simulink model "PIL_lqr_nl"  (R2024b)
settings: Solver=VariableStepAuto  StartTime=0.0  StopTime=params.simtime  RelTol=1e-3
values from neighbouring files (symbols this model uses):
  params = parameters()    [lqr_compare.m]    (also in lqr_main_isolated.m; lqr_pil.m)
undefined symbols (not defined in the file or in its folder): CR, LF, nl_model
libraries: instrumentseriallib x12
settings Model: Creator=ben83  LastModifiedBy=ben
settings RTWCC: GPUComputeCapability=3.5

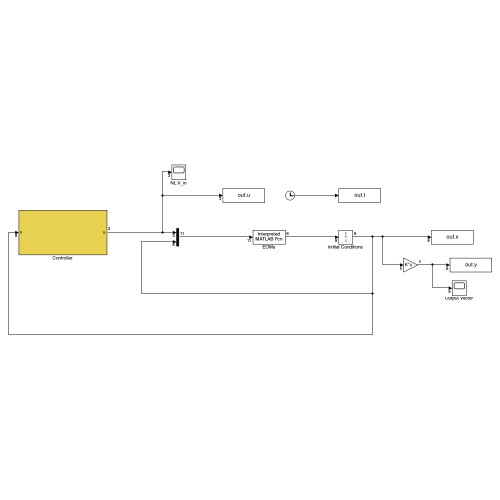
[thumbnail: Simulink's stored preview of the top-level diagram]
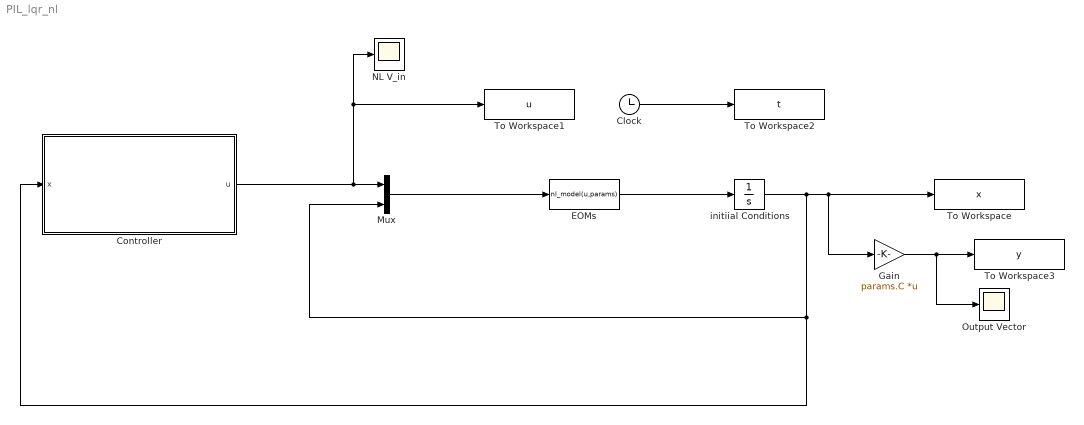
== system PIL_lqr_nl ==
  Clock : Clock
  Controller : Subsystem
  EOMs : MATLABFcn  MATLABFcn=nl_model(u,params)  OutputDimensions=8
  Gain : Gain  Gain=params.C  Multiplication=Matrix(K*u)
  Mux : Mux  Inputs=2
  NL V_in : Scope
  Output Vector : Scope
  To Workspace : ToWorkspace  VariableName=x  SampleTime=-1
  To Workspace1 : ToWorkspace  VariableName=u  SampleTime=-1
  To Workspace2 : ToWorkspace  VariableName=t  SampleTime=-1
  To Workspace3 : ToWorkspace  VariableName=y  SampleTime=-1
  initiial Conditions : Integrator  InitialCondition=params.ic
  wires:
  EOMs/1 -> initiial Conditions/1
  Mux/1 -> EOMs/1
  Clock/1 -> To Workspace2/1
  Controller/1(u) -> NL V_in/1, To Workspace1/1, Mux/1
  initiial Conditions/1 -> Controller/1(x), Mux/2, Gain/1, To Workspace/1
  Gain/1 -> Output Vector/1, To Workspace3/1

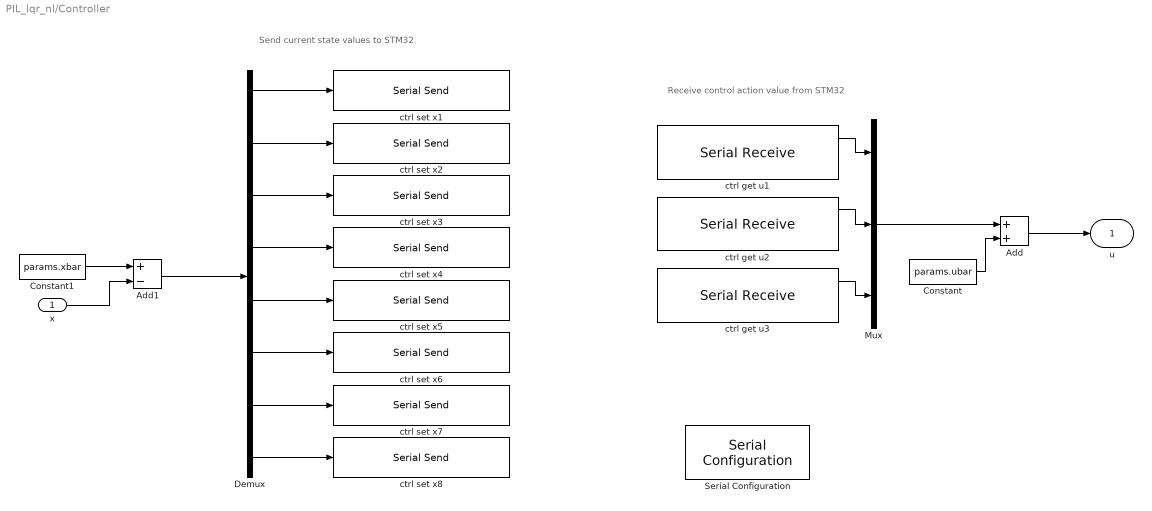
== system PIL_lqr_nl/Controller ==
  note: Send current state values to STM32
  note: Receive control action value from STM32
  x : Inport
  Add : Sum
  Add1 : Sum  Inputs=+-
  Constant : Constant  Value=params.ubar
  Constant1 : Constant  Value=params.xbar
  Demux : Demux  Outputs=8
  Mux : Mux  Inputs=3
  Serial Configuration : instrumentseriallib/Serial Configuration  Priority=-200000  PortSel=/dev/tty.usbmodem21103  Port=/dev/tty.usbmodem21103  ComPort=/dev/tty.usbmodem21103  BaudRate=921600  DataBits=8  Parity=none  StopBits=1  ByteOrder=little-endian  FlowControl=none  Timeout=10  SimulateUsing=Interpreted execution  BlockInModel=on  aMode=1
  ctrl get u1 : instrumentseriallib/Serial Receive  Priority=1  PortSel=/dev/tty.usbmodem21103  Port=/dev/tty.usbmodem21103  ComPort=/dev/tty.usbmodem21103  DataType=double  SaveDataType=uint8  ToggleHeader=off  Header=[]  ToggleDataSize=on  DataSize=[1 1]  ToggleTerminator=off  Terminator=<none>  CustomTerminator=[]  InputFormat=Column major  EnableBlockingMode=off  ActionDataUnavailable=Output custom value  ActionWhenDataUnavailable=Output custom value  CustomValue=0  SampleTime=0.01  SimulateUsing=Interpreted execution  BlockInModel=on  aMode=1
  ctrl get u2 : instrumentseriallib/Serial Receive  Priority=1  PortSel=/dev/tty.usbmodem21103  Port=/dev/tty.usbmodem21103  ComPort=/dev/tty.usbmodem21103  DataType=double  SaveDataType=uint8  ToggleHeader=off  Header=[]  ToggleDataSize=on  DataSize=[1 1]  ToggleTerminator=off  Terminator=<none>  CustomTerminator=[]  InputFormat=Column major  EnableBlockingMode=off  ActionDataUnavailable=Output custom value  ActionWhenDataUnavailable=Output custom value  CustomValue=0  SampleTime=0.01  SimulateUsing=Interpreted execution  BlockInModel=on  aMode=1
  ctrl get u3 : instrumentseriallib/Serial Receive  Priority=1  PortSel=/dev/tty.usbmodem21103  Port=/dev/tty.usbmodem21103  ComPort=/dev/tty.usbmodem21103  DataType=double  SaveDataType=uint8  ToggleHeader=off  Header=[]  ToggleDataSize=on  DataSize=[1 1]  ToggleTerminator=off  Terminator=<none>  CustomTerminator=[]  InputFormat=Column major  EnableBlockingMode=off  ActionDataUnavailable=Output custom value  ActionWhenDataUnavailable=Output custom value  CustomValue=0  SampleTime=0.01  SimulateUsing=Interpreted execution  BlockInModel=on  aMode=1
  ctrl set x{1..8} (8 alike) : instrumentseriallib/Serial Send  Priority=1  PortSel=/dev/tty.usbmodem21103  Port=/dev/tty.usbmodem21103  ComPort=/dev/tty.usbmodem21103  Header=[]  Terminator=CR/LF ('\r\n')  CustomTerminator=[]  EnableBlockingMode=off  SimulateUsing=Interpreted execution  BlockInModel=on  aMode=1
  u : Outport
  wires:
  Add1/1 -> Demux/1
  Mux/1 -> Add/1
  Constant1/1 -> Add1/1
  Constant/1 -> Add/2
  x/1 -> Add1/2
  Demux/1 -> ctrl set x1/1
  Demux/2 -> ctrl set x2/1
  Demux/3 -> ctrl set x3/1
  Demux/4 -> ctrl set x4/1
  Demux/8 -> ctrl set x8/1
  Demux/7 -> ctrl set x7/1
  Demux/6 -> ctrl set x6/1
  Demux/5 -> ctrl set x5/1
  ctrl get u1/1 -> Mux/1
  ctrl get u2/1 -> Mux/2
  ctrl get u3/1 -> Mux/3
  Add/1 -> u/1
